simulink model "kopter_se_zavazim_state_feedback"  (R2024b)
settings: Solver=ode4  StartTime=0.0  StopTime=16  FixedStep=0.01  RelTol=1e-3
values from neighbouring files (symbols this model uses):
  b_moment = 3.6e-7    (= 3.6e-07)    [parametry_kopter_se_zavazim.m]
  d = 1    [parametry_kopter_se_zavazim.m]
  g = 9.81    [parametry_kopter_se_zavazim.m]
  init_int_dref = -Ki\((Uinit-Us)+Kp*(Xinit_ss-Xs))    [odvozeni_stavova_regulace_a_LQR.m]
  init_int_ref = -Ki\(Kp*xss+uss)    [odvozeni_stavova_regulace_a_LQR.m]
  Ip = m*d^2    (= 1)    [parametry_kopter_se_zavazim.m]
  Ixx = 0.0222    [parametry_kopter_se_zavazim.m]
  Iyy = 0.0222    [parametry_kopter_se_zavazim.m]
  Izz = 0.0429    [parametry_kopter_se_zavazim.m]
  k_thrust = 9.3e-6    (= 9.3e-06)    [parametry_kopter_se_zavazim.m]
  Ki = K_ex_other_angles(:, 17:20)    [odvozeni_stavova_regulace_a_LQR.m]
  Kp = K_ex_other_angles(:, 1:16)    [odvozeni_stavova_regulace_a_LQR.m]
  l = 0.2051    [parametry_kopter_se_zavazim.m]
  L_obs = place(Ac', Cc', poles_obs)'    [odvozeni_stavova_regulace_a_LQR.m]
  M = 2    [parametry_kopter_se_zavazim.m]
  m = 1    [parametry_kopter_se_zavazim.m]
  Us = [(M+m)*g; 0; 0; 0]    [parametry_kopter_se_zavazim.m]
  Xinit_ss = [Xinit_matrix; [0 0 0 0 0 0 0 0]']    [parametry_kopter_se_zavazim.m]
  Xs = [0;0;0; 0;0;0; 0;0; 0;0;0; 0;0;0; 0;0]    [parametry_kopter_se_zavazim.m]
undefined symbols (not defined in the file or in its folder): L
libraries: simulink_extras x16
(part 1 of 4)
settings Model: Creator=Admin  LastModifiedBy=Admin

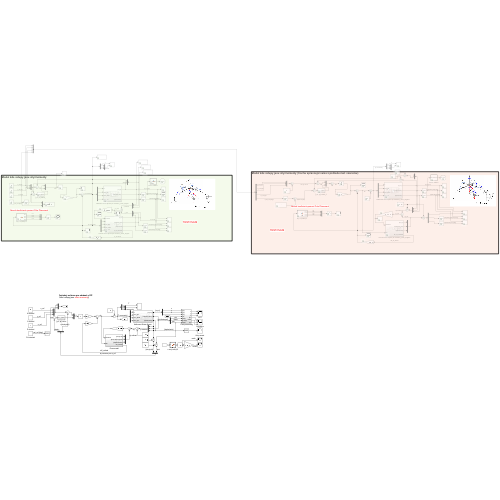
[thumbnail: Simulink's stored preview of the top-level diagram]
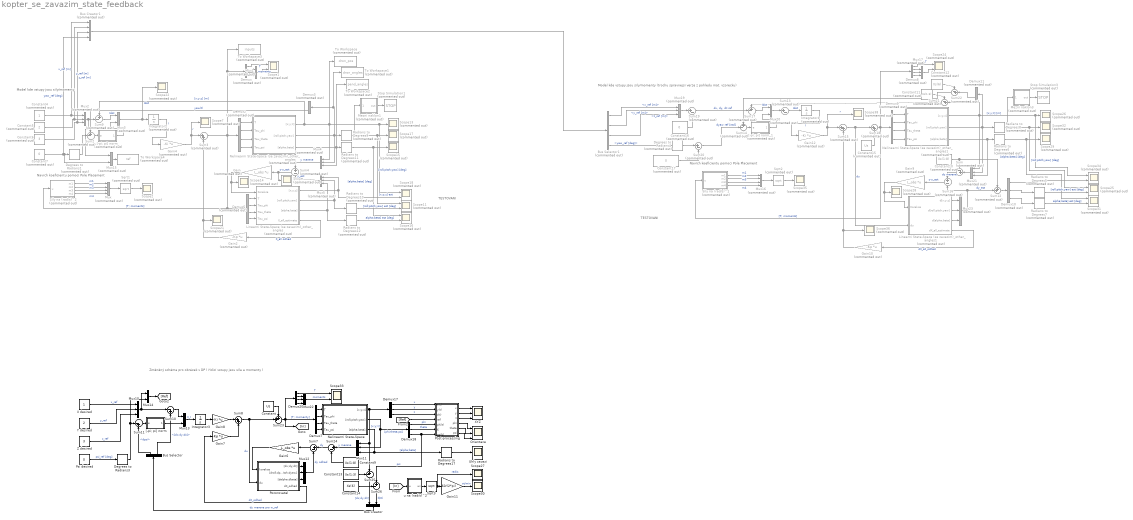
== system kopter_se_zavazim_state_feedback ==
  note: TESTOVANI
  note: Model kde vstupy jsou sily/momenty
  note: Navrch koeficientu pomoci Pole Placement
  note: Změněný schéma pro obrázek v DP
      | ( řídicí vstupy jsou síla a momenty )
  note: Model kde vstupy jsou sily/momenty (trochu spravnejsi verze z pohledu mat. vzorecku)
  note: Navrch koeficientu pomoci Pole Placement
  note: TESTOVANI
  Bus Creator : BusCreator  Inputs=2
  Bus Creator1 : BusCreator  Commented=on  Inputs=4
  Bus Selector : BusSelector  OutputSignals=dpsi,[dx;dy;dz]
  Bus Selector1 : BusSelector  Commented=on  OutputSignals=x_ref [m],y_ref [m],z_ref [m],yaw_ref [deg]
  Constant : Constant  Value=Us
  Constant10 : Constant  Commented=on  Value=Xs(1:8)
  Constant11 : Constant  Commented=on  Value=Xs(1:3)
  Constant12 : Constant  Commented=on  Value=Xs(6)
  Constant13 : Constant  Value=Xs(1:3)
  Constant14 : Constant  Value=Xs(6)
  Constant15 : Constant  Commented=on  Value=Us
  Constant16 : Constant  Commented=on  Value=0
  Constant17 : Constant  Commented=on  Value=0
  Constant4 : Constant  Commented=on
  Constant5 : Constant  Commented=on  Value=2
  Constant6 : Constant  Commented=on  Value=3
  Constant7 : Constant  Commented=on  Value=0
  Constant9 : Constant  Value=Xs(1:8)
  Degrees to Radians1 : simulink_extras/Transformations/Degrees to Radians  Commented=on
  Degrees to Radians3 : simulink_extras/Transformations/Degrees to Radians
  Degrees to Radians4 : simulink_extras/Transformations/Degrees to Radians  Commented=on
  Demux{,2,5,8..9} (5 alike) : Demux  Commented=on
  Demux10 : Demux  Commented=on  Outputs=3
  Demux11 : Demux  Commented=on  Outputs=3
  Demux17 : Demux  Outputs=3
  Demux18 : Demux  Outputs=3
  Demux20 : Demux
  Demux3 : Demux  Commented=on  Outputs=3
  Demux7 : Demux
  Gain : Gain  Commented=on  Gain=L_obs  Multiplication=Matrix(K*u)
  Gain10 : Gain  Commented=on  Gain=-Kp  Multiplication=Matrix(K*u)
  Gain11 : Gain  Gain=60/(2*pi)
  Gain12 : Gain  Commented=on  Gain=-Ki  Multiplication=Matrix(K*u)
  Gain2 : Gain  Commented=on  Gain=-Kp  Multiplication=Matrix(K*u)
  Gain4 : Gain  Commented=on  Gain=-Ki  Multiplication=Matrix(K*u)
  Gain6 : Gain  Gain=L_obs  Multiplication=Matrix(K*u)
  Gain7 : Gain  Gain=-Kp  Multiplication=Matrix(K*u)
  Gain8 : Gain  Gain=-Ki  Multiplication=Matrix(K*u)
  Gain9 : Gain  Commented=on  Gain=L_obs  Multiplication=Matrix(K*u)
  Integrator1 : Integrator  Commented=on  InitialCondition=init_int_ref
  Integrator3 : Integrator  InitialCondition=init_int_dref
  Integrator4 : Integrator  Commented=on  InitialCondition=init_int_dref
  Linearni State-Space (se zavazim)_other_angles : Subsystem  Commented=on
  Linearni State-Space (se zavazim)_other_angles1 : Subsystem  Commented=on
  Mezni naklon1 : MATLAB Function  Commented=on  TreatAsAtomicUnit=on
  Mezni naklon3 : MATLAB Function  Commented=on  TreatAsAtomicUnit=on
  Mux : Mux  Commented=on
  Mux{1..2,4..5,17,19,21,23} (8 alike) : Mux  Commented=on  Inputs=3
  Mux{10..12,22} (4 alike) : Mux  Inputs=3
  Mux13 : Mux  Inputs=2
  Mux14 : Mux  Inputs=2
  Mux15 : Mux  Commented=on  Inputs=2
  Mux16 : Mux  Commented=on
  Mux20 : Mux  Commented=on  Inputs=2
  Mux3 : Mux  Commented=on  Inputs=2
  Nelinearni State-Space : Subsystem
  Nelinearni State-Space (se zavazim)_other_angles : Subsystem  Commented=on
  Nelinearni State-Space (se zavazim)_other_angles1 : Subsystem  Commented=on
  Orientace : Scope  NumInputPorts=3
  Post-processing : Subsystem
  Pozorovatel : Subsystem
  Psi desired : Constant  Value=0
  Radians to Degrees{5..12} (8 alike) : simulink_extras/Transformations/Radians to Degrees  Commented=on
  Radians to Degrees17 : simulink_extras/Transformations/Radians to Degrees
  Scope{,2,7,13..15,17,21..22,26,28..29,32,35..36,38} (16 alike) : Scope  Commented=on
  Scope{1,11,16,18,24..25,31,34} (8 alike) : Scope  Commented=on  NumInputPorts=2
  Scope27 : Scope
  Scope30 : Scope
  Scope33 : Scope  NumInputPorts=2
  Sily na (rad/s)^1 : MATLAB Function  Commented=on  TreatAsAtomicUnit=on
  Sily na (rad/s)^2 : MATLAB Function  Commented=on  TreatAsAtomicUnit=on
  Sqrt1 : Sqrt  Commented=on
  Sqrt2 : Sqrt  Commented=on
  Sqrt3 : Sqrt
  Stop Simulation1 : Stop  Commented=on
  Stop Simulation3 : Stop  Commented=on
  Sum : Sum  Commented=on  Inputs=-+|
  Sum10 : Sum  Inputs=|-+
  Sum11 : Sum  Inputs=|-+
  Sum12 : Sum  Commented=on  Inputs=++|
  Sum13 : Sum  Commented=on  Inputs=|+-
  Sum{2,9,14,17} (4 alike) : Sum  Commented=on  Inputs=+-|
  Sum15 : Sum  Commented=on  Inputs=|++
  Sum16 : Sum  Commented=on  Inputs=+|-
  Sum18 : Sum  Commented=on  Inputs=|++
  Sum19 : Sum  Commented=on  Inputs=|+-
  Sum20 : Sum  Commented=on  Inputs=|+-
  Sum21 : Sum  Commented=on  Inputs=-+|
  Sum22 : Sum  Commented=on  Inputs=-+|
  Sum23 : Sum  Inputs=++|
  Sum24 : Sum  Inputs=|+-
  Sum25 : Sum  Inputs=-+|
  Sum26 : Sum  Inputs=-+|
  Sum3 : Sum  Commented=on  Inputs=|++
  Sum4 : Sum  Commented=on  Inputs=+|-
  Sum7 : Sum  Inputs=|+-
  Sum8 : Sum  Inputs=|++
  To Workspace : ToWorkspace  Commented=on  VariableName=dron_pos  SaveFormat=Timeseries  SampleTime=-1
  To Workspace1 : ToWorkspace  Commented=on  VariableName=dron_angles  SaveFormat=Timeseries  SampleTime=-1
  To Workspace2 : ToWorkspace  Commented=on  VariableName=pend_angles  SaveFormat=Timeseries  SampleTime=-1
  To Workspace3 : ToWorkspace  Commented=on  VariableName=inputs  SaveFormat=Timeseries  SampleTime=-1
  To Workspace4 : ToWorkspace  Commented=on  VariableName=ref  SaveFormat=Timeseries  SampleTime=-1
  Uhly zavazi : Scope
  X desired : Constant
  XYZ : Scope  NumInputPorts=3
  Y desired : Constant  Value=2
  Z desired : Constant  Value=3
  "[-pi; pi] norm" : Subsystem
  "[-pi; pi] norm_" : Subsystem  Commented=on
  "[-pi; pi] norm_1" : Subsystem  Commented=on
  u na (rad/s)^2 : MATLAB Function  TreatAsAtomicUnit=on
  wires:
  Linearni State-Space (se zavazim)_other_angles/1("[x;y;z]") -> Mux5/1, Scope18/2  "[x;y;z] est"
  Demux5/3 -> Linearni State-Space (se zavazim)_other_angles/4(Tau_theta)
  Demux5/2 -> Linearni State-Space (se zavazim)_other_angles/3(Tau_phi)
  Nelinearni State-Space (se zavazim)_other_angles/3("[alpha;beta]") -> To Workspace2/1, Mux4/3, Radians to Degrees11/1
  Linearni State-Space (se zavazim)_other_angles/3("[alpha;beta]") -> Radians to Degrees12/1, Mux5/3
  Radians to Degrees10/1 -> Scope11/2  "[roll;pitch;yaw] est [deg]"
  Linearni State-Space (se zavazim)_other_angles/2("[roll;pitch;yaw]") -> Mux5/2, Radians to Degrees10/1
  Radians to Degrees12/1 -> Scope16/2  "alpha;beta] est [deg]"
  Demux5/1 -> Linearni State-Space (se zavazim)_other_angles/2(T)
  Demux5/4 -> Linearni State-Space (se zavazim)_other_angles/5(Tau_psi)
  Radians to Degrees9/1 -> Scope11/1, Scope17/1, Mezni naklon1/1(angles)  "[roll;pitch;yaw] [deg]"
  Radians to Degrees11/1 -> Scope16/1, Scope15/1  "[alpha;beta] [deg]"
  Demux2/3 -> Nelinearni State-Space (se zavazim)_other_angles/3(Tau_theta)
  Demux2/2 -> Nelinearni State-Space (se zavazim)_other_angles/2(Tau_phi)
  Constant5/1 -> Bus Creator1/2, Mux2/2  "y_ref [m]"
  Constant7/1 -> Bus Creator1/4, Mux15/2, Degrees to Radians1/1  "yaw_ref [deg]"
  Constant6/1 -> Bus Creator1/3, Mux2/3  "z_ref [m]"
  Gain2/1 -> Scope21/1, Sum3/2
  Degrees to Radians1/1 -> Sum2/2
  Sum3/1 -> Sily na (rad/s)^2/1(u), Demux5/1, To Workspace3/1, Demux/1, Demux2/1  "[T; moments]"
  Demux2/4 -> Nelinearni State-Space (se zavazim)_other_angles/4(Tau_psi)
  Gain4/1 -> Scope7/1, Sum3/1  "r"
  Demux2/1 -> Nelinearni State-Space (se zavazim)_other_angles/1(T)
  Integrator1/1 -> Gain4/1  "I"
  Constant4/1 -> Bus Creator1/1, Mux2/1  "x_ref [m]"
  Demux3/3 -> Sum2/1  "yaw(t)"
  Nelinearni State-Space (se zavazim)_other_angles/1("[x;y;z]") -> Sum9/1, To Workspace/1, Mux4/1, Scope18/1, Scope13/1  "[x;y;z] [m]"
  Nelinearni State-Space (se zavazim)_other_angles/2("[roll;pitch;yaw]") -> To Workspace1/1, Demux3/1, Radians to Degrees9/1, Mux4/2
  Mezni naklon1/1(out) -> Stop Simulation1/1
  Linearni State-Space (se zavazim)_other_angles/4(X_all_estimate) -> Gain2/1  "X_all odhad"
  Gain/1 -> Scope14/1, Linearni State-Space (se zavazim)_other_angles/1(Korekce)
  Sum4/1 -> Scope/1, Gain/1  "y-y_est"
  Mux5/1 -> Sum4/2  "y_est"
  Sily na (rad/s)^2/4(m4) -> Mux/4  "m4"
  Sily na (rad/s)^2/2(m2) -> Mux/2  "m2"
  Sily na (rad/s)^2/1(m1) -> Mux/1  "m1"
  Sily na (rad/s)^2/3(m3) -> Mux/3  "m3"
  Mux/1 -> Sqrt1/1
  Mux4/1 -> Sum4/1  "y merene"
  Demux/1 -> Scope1/1  "T"
  Demux/2 -> Mux1/1
  Demux/3 -> Mux1/2
  Demux/4 -> Mux1/3
  Mux1/1 -> Scope1/2  "moments"
  X desired/1 -> Mux10/1  "x_ref"
  Y desired/1 -> Mux10/2  "y_ref"
  Z desired/1 -> Mux10/3  "z_ref"
  Psi desired/1 -> Degrees to Radians3/1  "psi_ref [deg]"
  Degrees to Radians3/1 -> Mux14/2, Sum11/1
  Demux7/1 -> Nelinearni State-Space/1(T)
  Demux7/2 -> Nelinearni State-Space/2(Tau_phi)
  Demux7/3 -> Nelinearni State-Space/3(Tau_theta)
  Demux7/4 -> Nelinearni State-Space/4(Tau_psi)
  Nelinearni State-Space/2("[roll;pitch;yaw]") -> Demux18/1, Mux11/2  "[phi;theta;psi]"
  Demux17/2 -> Post-processing/2(y(t))  "y"
  Nelinearni State-Space/1("[x;y;z]") -> Demux17/1, Sum25/2, Mux11/1  "[x;y;z]"
  Demux17/3 -> Post-processing/3(z(t))  "z"
  Nelinearni State-Space/3("[alpha;beta]") -> Radians to Degrees17/1, Mux11/3  "[alpha;beta]"
  Post-processing/3(z) -> XYZ/3
  Post-processing/2(y) -> XYZ/2
  Post-processing/1(x) -> XYZ/1
  Demux18/2 -> Post-processing/6(theta(t))  "theta"
  Radians to Degrees17/1 -> Uhly zavazi/1
  [Ref] -> Post-processing/4(ref)
  Post-processing/6(psi) -> Orientace/3
  Demux18/1 -> Post-processing/5(phi(t))  "phi"
  Demux18/3 -> Post-processing/7(psi(t)), Sum26/2  "psi"
  Post-processing/4(phi) -> Orientace/1
  Post-processing/5(theta) -> Orientace/2
  Demux17/1 -> Post-processing/1(x(t))  "x"
  Mux11/1 -> Sum24/1  "y merene"
  Pozorovatel/1("[dx;dy;dz]") -> Mux12/1
  Pozorovatel/2("[droll;dpitch;dyaw]") -> Mux12/2
  Pozorovatel/3("[dalpha;dbeta]") -> Mux12/3
  Mux12/1 -> Sum7/2  "dy odhad"
  Sum7/1 -> Gain6/1
  Gain6/1 -> Pozorovatel/1(korekce)
  Sum23/1 -> [In], Demux7/1, Demux20/1  "[T; momenty]"
  Integrator3/1 -> Gain8/1
  Gain8/1 -> Sum8/1
  Pozorovatel/4(dX_odhad) -> Gain7/1  "dX_odhad"
  Gain7/1 -> Sum8/2
  Demux20/2 -> Mux22/1
  Demux20/3 -> Mux22/2
  Demux20/1 -> Scope33/1  "T"
  Mux22/1 -> Scope33/2  "moments"
  Demux20/4 -> Mux22/3
  Bus Creator/1 -> Bus Selector/1  "dy merene pro w_ref"
  Sqrt1/1 -> Scope2/1
  Bus Selector/2 -> Sum10/2  "<[dx;dy;dz]>"
  Bus Selector/1 -> Sum11/2  "<dpsi>"
  Sqrt3/1 -> Gain11/1, Scope27/1  "rad/s"
  Gain11/1 -> Scope30/1  "ot/min"
  u na (rad/s)^2/1(wi) -> Sqrt3/1
  [In] -> u na (rad/s)^2/1(u)
  Mux2/1 -> Mux15/1, Sum9/2
  Sum2/1 -> "[-pi; pi] norm_"/1(e)
  Sum9/1 -> Mux3/1  "Idot"
  "[-pi; pi] norm_"/1(e_norm) -> Mux3/2
  Mux10/1 -> Mux14/1, Sum10/1
  Sum11/1 -> "[-pi; pi] norm"/1(e)
  Sum10/1 -> Mux13/1
  "[-pi; pi] norm"/1(e_norm) -> Mux13/2
  Mux13/1 -> Integrator3/1  "X_I"
  Mux14/1 -> [Ref]
  Mux3/1 -> Scope22/1, Integrator1/1  "Idot"
  Mux15/1 -> To Workspace4/1
  Bus Selector1/2 -> Mux19/2  "<y_ref [m]>"
  Nelinearni State-Space (se zavazim)_other_angles1/2("[roll;pitch;yaw]") -> Demux11/1, Mux21/2, Radians to Degrees8/1
  Radians to Degrees8/1 -> Scope25/1, Scope32/1, Mezni naklon3/1(angles)  "[roll;pitch;yaw] [deg]"
  Mux23/1 -> Sum12/2, Sum16/2  "dy_est"
  Sqrt2/1 -> Scope35/1
  Bus Selector1/4 -> Degrees to Radians4/1  "<yaw_ref [deg]>"
  Sum16/1 -> Gain9/1  "y-y_est"
  Bus Selector1/1 -> Mux19/1  "<x_ref [m]>"
  Sum14/1 -> "[-pi; pi] norm_1"/1(e)
  Sily na (rad/s)^1/2(m2) -> Mux16/2  "m2"
  Radians to Degrees5/1 -> Scope25/2  "[roll;pitch;yaw] est [deg]"
  Mux19/1 -> Sum19/1
  Mux20/1 -> Sum13/1
  Degrees to Radians4/1 -> Sum20/1
  Nelinearni State-Space (se zavazim)_other_angles1/3("[alpha;beta]") -> Mux21/3, Radians to Degrees6/1
  Bus Selector1/3 -> Mux19/3  "<z_ref [m]>"
  Mux16/1 -> Sqrt2/1
  Sily na (rad/s)^1/1(m1) -> Mux16/1  "m1"
  Linearni State-Space (se zavazim)_other_angles1/1(d[x;y;z]) -> Mux23/1
  Linearni State-Space (se zavazim)_other_angles1/4(dX_all_estimate) -> Gain10/1  "dX_all_odhad"
  Radians to Degrees7/1 -> Scope31/2  "alpha;beta] est [deg]"
  Demux9/3 -> Nelinearni State-Space (se zavazim)_other_angles1/3(Tau_theta)
  Gain9/1 -> Scope28/1, Linearni State-Space (se zavazim)_other_angles1/1(Korekce)
  Radians to Degrees6/1 -> Scope31/1, Scope29/1  "[alpha;beta] [deg]"
  Integrator4/1 -> Gain12/1  "I"
  Demux9/2 -> Nelinearni State-Space (se zavazim)_other_angles1/2(Tau_phi)
  Mezni naklon3/1(out) -> Stop Simulation3/1
  "[-pi; pi] norm_1"/1(e_norm) -> Mux20/2
  Sily na (rad/s)^1/3(m3) -> Mux16/3  "m3"
  Gain12/1 -> Sum15/1, Scope38/1  "r"
  Sum/1 -> Sum16/1  "dy merene"
  Sum17/1 -> Mux20/1  "Idot"
  Linearni State-Space (se zavazim)_other_angles1/3(d[alpha;beta]) -> Mux23/3
  Sum13/1 -> Integrator4/1  "Idot"
  Demux9/1 -> Nelinearni State-Space (se zavazim)_other_angles1/1(T)
  Linearni State-Space (se zavazim)_other_angles1/2(d[roll;pitch;yaw]) -> Mux23/2
  Demux9/4 -> Nelinearni State-Space (se zavazim)_other_angles1/4(Tau_psi)
  Sily na (rad/s)^1/4(m4) -> Mux16/4  "m4"
  Constant15/1 -> Sum18/2
  Demux8/4 -> Mux17/3
  Mux17/1 -> Scope24/2
  Demux8/3 -> Mux17/2
  Demux8/1 -> Scope24/1  "T"
  Sum18/1 -> Demux8/1, Sily na (rad/s)^1/1(u), Demux9/1  "[T; moments]"
  Demux8/2 -> Mux17/1
  Gain10/1 -> Sum15/2, Scope36/1
  Sum15/1 -> Linearni State-Space (se zavazim)_other_angles1/2(du), Sum18/1  "du"
  Sum19/1 -> Sum17/2  "dx, dy, dz ref"
  Constant16/1 -> Sum19/2
  Constant17/1 -> Sum20/2
  Sum20/1 -> Sum14/2  "dyaw ref [rad]"
  Nelinearni State-Space (se zavazim)_other_angles1/1("[x;y;z]") -> Sum21/2, Mux21/1, Scope34/1, Scope26/1  "[x;y;z] [m]"
  Bus Creator1/1 -> Bus Selector1/1
  Mux21/1 -> Sum/2
  Constant10/1 -> Sum12/1, Sum/1
  Sum12/1 -> Demux10/1
  Demux10/1 -> Scope34/2
  Demux10/2 -> Radians to Degrees5/1
  Demux10/3 -> Radians to Degrees7/1
  Sum21/1 -> Sum17/1
  Constant11/1 -> Sum21/1
  Sum22/1 -> Sum14/1
  Constant12/1 -> Sum22/1
  Demux11/3 -> Sum22/2
  Sum8/1 -> Sum23/2, Pozorovatel/2(du)  "du"
  Constant/1 -> Sum23/1
  Sum24/1 -> Sum7/1  "dy"
  Constant9/1 -> Sum24/2
  Sum25/1 -> Bus Creator/1  "[dx;dy;dz]"
  Constant13/1 -> Sum25/1
  Sum26/1 -> Bus Creator/2  "dpsi"
  Constant14/1 -> Sum26/1

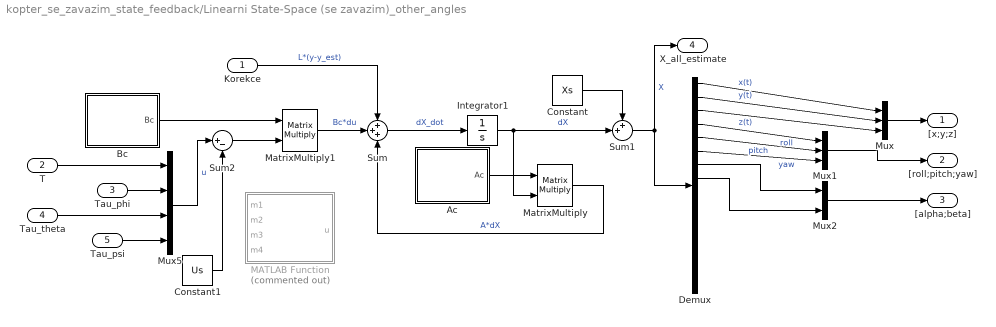
== system kopter_se_zavazim_state_feedback/Linearni State-Space (se zavazim)_other_angles ==
  Korekce : Inport
  T : Inport  Port=2
  Tau_phi : Inport  Port=3
  Tau_theta : Inport  Port=4
  Tau_psi : Inport  Port=5
  Ac : MATLAB Function  TreatAsAtomicUnit=on
  Bc : MATLAB Function  TreatAsAtomicUnit=on
  Constant : Constant  Value=Xs
  Constant1 : Constant  Value=Us
  Demux : Demux  Outputs=16
  Integrator1 : Integrator  InitialCondition=Xinit_ss - Xs
  MATLAB Function : MATLAB Function  Commented=on  TreatAsAtomicUnit=on
  MatrixMultiply : Product  Multiplication=Matrix(*)
  MatrixMultiply1 : Product  Multiplication=Matrix(*)
  Mux : Mux  Inputs=3
  Mux1 : Mux  Inputs=3
  Mux2 : Mux  Inputs=2
  Mux5 : Mux
  Sum : Sum  Inputs=+++
  Sum1 : Sum  Inputs=++|
  Sum2 : Sum  Inputs=|+-
  "[x;y;z]" : Outport
  "[roll;pitch;yaw]" : Outport  Port=2
  "[alpha;beta]" : Outport  Port=3
  X_all_estimate : Outport  Port=4
  wires:
  Mux5/1 -> Sum2/1  "u"
  Ac/1(Ac) -> MatrixMultiply/1
  Integrator1/1 -> Sum1/2, MatrixMultiply/2  "dX"
  Demux/1 -> Mux/1  "x(t)"
  Demux/2 -> Mux/2  "y(t)"
  Demux/3 -> Mux/3  "z(t)"
  Mux/1 -> "[x;y;z]"/1
  Demux/4 -> Mux1/1  "roll"
  Demux/5 -> Mux1/2  "pitch"
  Demux/6 -> Mux1/3  "yaw"
  Mux1/1 -> "[roll;pitch;yaw]"/1
  Sum/1 -> Integrator1/1  "dX_dot"
  MatrixMultiply1/1 -> Sum/2  "Bc*du"
  MatrixMultiply/1 -> Sum/3  "A*dX"
  Bc/1(Bc) -> MatrixMultiply1/1
  Sum1/1 -> Demux/1, X_all_estimate/1  "X"
  Constant/1 -> Sum1/1
  Constant1/1 -> Sum2/2
  Sum2/1 -> MatrixMultiply1/2
  Mux2/1 -> "[alpha;beta]"/1
  Demux/7 -> Mux2/1
  Demux/8 -> Mux2/2
  Tau_psi/1 -> Mux5/4
  T/1 -> Mux5/1
  Tau_theta/1 -> Mux5/3
  Tau_phi/1 -> Mux5/2
  Korekce/1 -> Sum/1  "L*(y-y_est)"

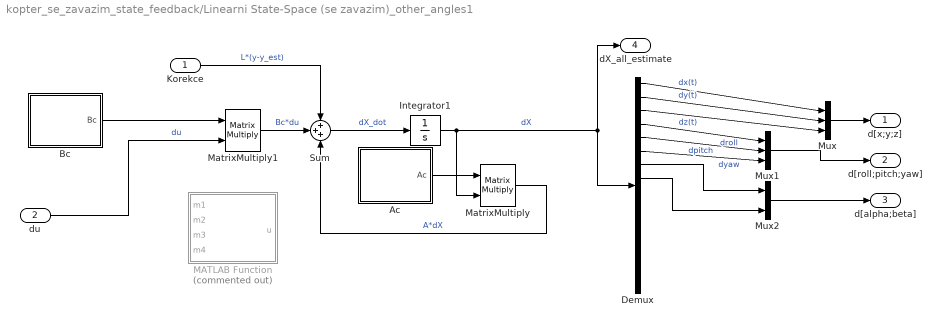
== system kopter_se_zavazim_state_feedback/Linearni State-Space (se zavazim)_other_angles1 ==
  Korekce : Inport
  du : Inport  Port=2
  Ac : MATLAB Function  TreatAsAtomicUnit=on
  Bc : MATLAB Function  TreatAsAtomicUnit=on
  Demux : Demux  Outputs=16
  Integrator1 : Integrator  InitialCondition=Xinit_ss - Xs
  MATLAB Function : MATLAB Function  Commented=on  TreatAsAtomicUnit=on
  MatrixMultiply : Product  Multiplication=Matrix(*)
  MatrixMultiply1 : Product  Multiplication=Matrix(*)
  Mux : Mux  Inputs=3
  Mux1 : Mux  Inputs=3
  Mux2 : Mux  Inputs=2
  Sum : Sum  Inputs=+++
  d[x;y;z] : Outport
  d[roll;pitch;yaw] : Outport  Port=2
  d[alpha;beta] : Outport  Port=3
  dX_all_estimate : Outport  Port=4
  wires:
  du/1 -> MatrixMultiply1/2  "du"
  Ac/1(Ac) -> MatrixMultiply/1
  Integrator1/1 -> Demux/1, dX_all_estimate/1, MatrixMultiply/2  "dX"
  Demux/1 -> Mux/1  "dx(t)"
  Demux/2 -> Mux/2  "dy(t)"
  Demux/3 -> Mux/3  "dz(t)"
  Mux/1 -> d[x;y;z]/1
  Demux/4 -> Mux1/1  "droll"
  Demux/5 -> Mux1/2  "dpitch"
  Demux/6 -> Mux1/3  "dyaw"
  Mux1/1 -> d[roll;pitch;yaw]/1
  Sum/1 -> Integrator1/1  "dX_dot"
  MatrixMultiply1/1 -> Sum/2  "Bc*du"
  MatrixMultiply/1 -> Sum/3  "A*dX"
  Bc/1(Bc) -> MatrixMultiply1/1
  Mux2/1 -> d[alpha;beta]/1
  Demux/7 -> Mux2/1
  Demux/8 -> Mux2/2
  Korekce/1 -> Sum/1  "L*(y-y_est)"

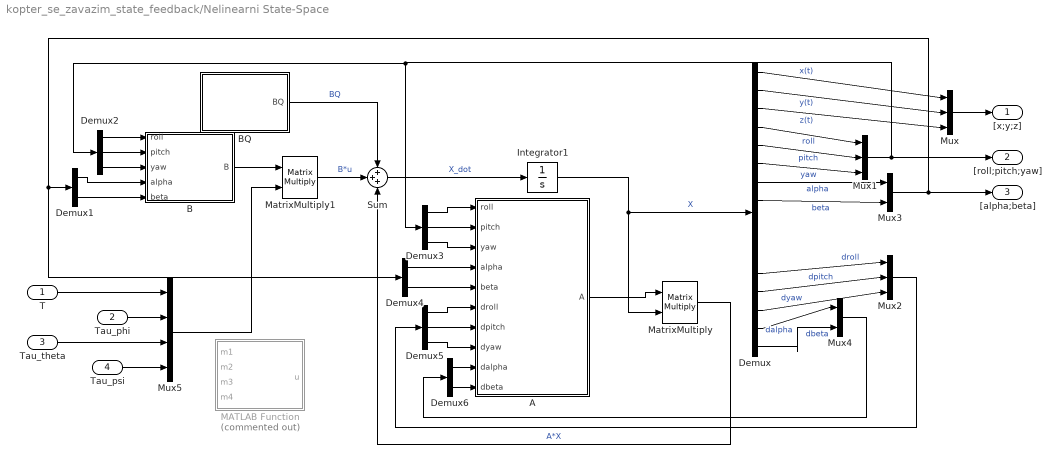
== system kopter_se_zavazim_state_feedback/Nelinearni State-Space ==
  T : Inport
  Tau_phi : Inport  Port=2
  Tau_theta : Inport  Port=3
  Tau_psi : Inport  Port=4
  A : MATLAB Function  TreatAsAtomicUnit=on
  B : MATLAB Function  TreatAsAtomicUnit=on
  BQ : MATLAB Function  TreatAsAtomicUnit=on
  Demux : Demux  Outputs=16
  Demux1 : Demux  Outputs=2
  Demux2 : Demux  Outputs=3
  Demux3 : Demux  Outputs=3
  Demux4 : Demux  Outputs=2
  Demux5 : Demux  Outputs=3
  Demux6 : Demux  Outputs=2
  Integrator1 : Integrator  InitialCondition=Xinit_ss
  MATLAB Function : MATLAB Function  Commented=on  TreatAsAtomicUnit=on
  MatrixMultiply : Product  Multiplication=Matrix(*)
  MatrixMultiply1 : Product  Multiplication=Matrix(*)
  Mux : Mux  Inputs=3
  Mux1 : Mux  Inputs=3
  Mux2 : Mux  Inputs=3
  Mux3 : Mux  Inputs=2
  Mux4 : Mux  Inputs=2
  Mux5 : Mux
  Sum : Sum  Inputs=+++
  "[x;y;z]" : Outport
  "[roll;pitch;yaw]" : Outport  Port=2
  "[alpha;beta]" : Outport  Port=3
  wires:
  A/1(A) -> MatrixMultiply/1
  Integrator1/1 -> MatrixMultiply/2, Demux/1  "X"
  Demux/1 -> Mux/1  "x(t)"
  Demux/2 -> Mux/2  "y(t)"
  Demux/3 -> Mux/3  "z(t)"
  Mux/1 -> "[x;y;z]"/1
  Demux/4 -> Mux1/1  "roll"
  Demux/5 -> Mux1/2  "pitch"
  Demux/6 -> Mux1/3  "yaw"
  Mux1/1 -> Demux2/1, Demux3/1, "[roll;pitch;yaw]"/1
  Demux/12 -> Mux2/1  "droll"
  Demux/13 -> Mux2/2  "dpitch"
  Demux/14 -> Mux2/3  "dyaw"
  Demux2/1 -> B/1(roll)
  Demux2/2 -> B/2(pitch)
  Demux2/3 -> B/3(yaw)
  Demux3/2 -> A/2(pitch)
  Demux3/1 -> A/1(roll)
  Demux3/3 -> A/3(yaw)
  Demux5/2 -> A/7(dpitch)
  Demux5/1 -> A/6(droll)
  Demux5/3 -> A/8(dyaw)
  Sum/1 -> Integrator1/1  "X_dot"
  BQ/1(BQ) -> Sum/1  "BQ"
  MatrixMultiply1/1 -> Sum/2  "B*u"
  B/1(B) -> MatrixMultiply1/1
  MatrixMultiply/1 -> Sum/3  "A*X"
  Mux2/1 -> Demux5/1
  Demux/7 -> Mux3/1  "alpha"
  Demux/8 -> Mux3/2  "beta"
  Mux3/1 -> Demux4/1, Demux1/1, "[alpha;beta]"/1
  Demux1/2 -> B/5(beta)
  Demux1/1 -> B/4(alpha)
  Demux4/2 -> A/5(beta)
  Demux4/1 -> A/4(alpha)
  Demux/15 -> Mux4/1  "dalpha"
  Demux/16 -> Mux4/2  "dbeta"
  Demux6/1 -> A/9(dalpha)
  Demux6/2 -> A/10(dbeta)
  Mux4/1 -> Demux6/1
  Tau_theta/1 -> Mux5/3
  Tau_psi/1 -> Mux5/4
  Tau_phi/1 -> Mux5/2
  Mux5/1 -> MatrixMultiply1/2
  T/1 -> Mux5/1

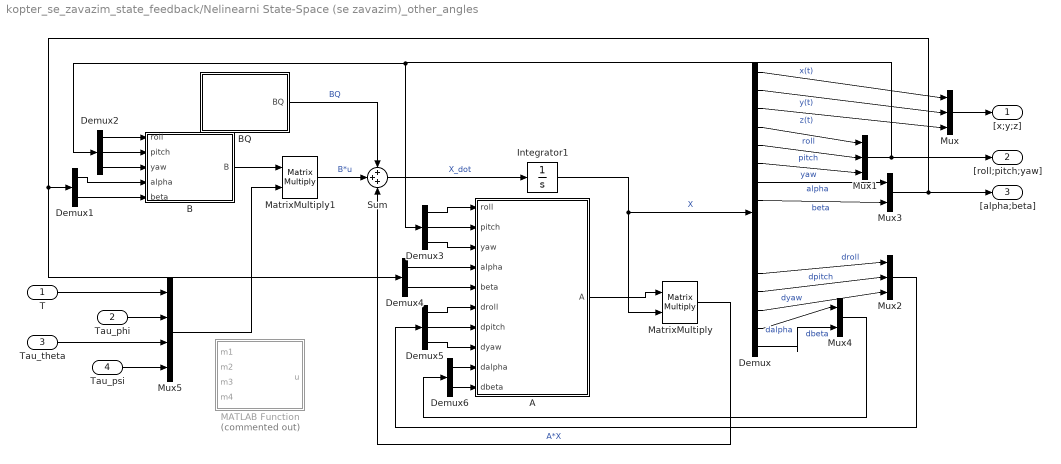
== system kopter_se_zavazim_state_feedback/Nelinearni State-Space (se zavazim)_other_angles ==
  T : Inport
  Tau_phi : Inport  Port=2
  Tau_theta : Inport  Port=3
  Tau_psi : Inport  Port=4
  A : MATLAB Function  TreatAsAtomicUnit=on
  B : MATLAB Function  TreatAsAtomicUnit=on
  BQ : MATLAB Function  TreatAsAtomicUnit=on
  Demux : Demux  Outputs=16
  Demux1 : Demux  Outputs=2
  Demux2 : Demux  Outputs=3
  Demux3 : Demux  Outputs=3
  Demux4 : Demux  Outputs=2
  Demux5 : Demux  Outputs=3
  Demux6 : Demux  Outputs=2
  Integrator1 : Integrator  InitialCondition=Xinit_ss
  MATLAB Function : MATLAB Function  Commented=on  TreatAsAtomicUnit=on
  MatrixMultiply : Product  Multiplication=Matrix(*)
  MatrixMultiply1 : Product  Multiplication=Matrix(*)
  Mux : Mux  Inputs=3
  Mux1 : Mux  Inputs=3
  Mux2 : Mux  Inputs=3
  Mux3 : Mux  Inputs=2
  Mux4 : Mux  Inputs=2
  Mux5 : Mux
  Sum : Sum  Inputs=+++
  "[x;y;z]" : Outport
  "[roll;pitch;yaw]" : Outport  Port=2
  "[alpha;beta]" : Outport  Port=3
  wires:
  A/1(A) -> MatrixMultiply/1
  Integrator1/1 -> MatrixMultiply/2, Demux/1  "X"
  Demux/1 -> Mux/1  "x(t)"
  Demux/2 -> Mux/2  "y(t)"
  Demux/3 -> Mux/3  "z(t)"
  Mux/1 -> "[x;y;z]"/1
  Demux/4 -> Mux1/1  "roll"
  Demux/5 -> Mux1/2  "pitch"
  Demux/6 -> Mux1/3  "yaw"
  Mux1/1 -> Demux2/1, Demux3/1, "[roll;pitch;yaw]"/1
  Demux/12 -> Mux2/1  "droll"
  Demux/13 -> Mux2/2  "dpitch"
  Demux/14 -> Mux2/3  "dyaw"
  Demux2/1 -> B/1(roll)
  Demux2/2 -> B/2(pitch)
  Demux2/3 -> B/3(yaw)
  Demux3/2 -> A/2(pitch)
  Demux3/1 -> A/1(roll)
  Demux3/3 -> A/3(yaw)
  Demux5/2 -> A/7(dpitch)
  Demux5/1 -> A/6(droll)
  Demux5/3 -> A/8(dyaw)
  Sum/1 -> Integrator1/1  "X_dot"
  BQ/1(BQ) -> Sum/1  "BQ"
  MatrixMultiply1/1 -> Sum/2  "B*u"
  B/1(B) -> MatrixMultiply1/1
  MatrixMultiply/1 -> Sum/3  "A*X"
  Mux2/1 -> Demux5/1
  Demux/7 -> Mux3/1  "alpha"
  Demux/8 -> Mux3/2  "beta"
  Mux3/1 -> Demux4/1, Demux1/1, "[alpha;beta]"/1
  Demux1/2 -> B/5(beta)
  Demux1/1 -> B/4(alpha)
  Demux4/2 -> A/5(beta)
  Demux4/1 -> A/4(alpha)
  Demux/15 -> Mux4/1  "dalpha"
  Demux/16 -> Mux4/2  "dbeta"
  Demux6/1 -> A/9(dalpha)
  Demux6/2 -> A/10(dbeta)
  Mux4/1 -> Demux6/1
  Tau_theta/1 -> Mux5/3
  Tau_psi/1 -> Mux5/4
  Tau_phi/1 -> Mux5/2
  Mux5/1 -> MatrixMultiply1/2
  T/1 -> Mux5/1

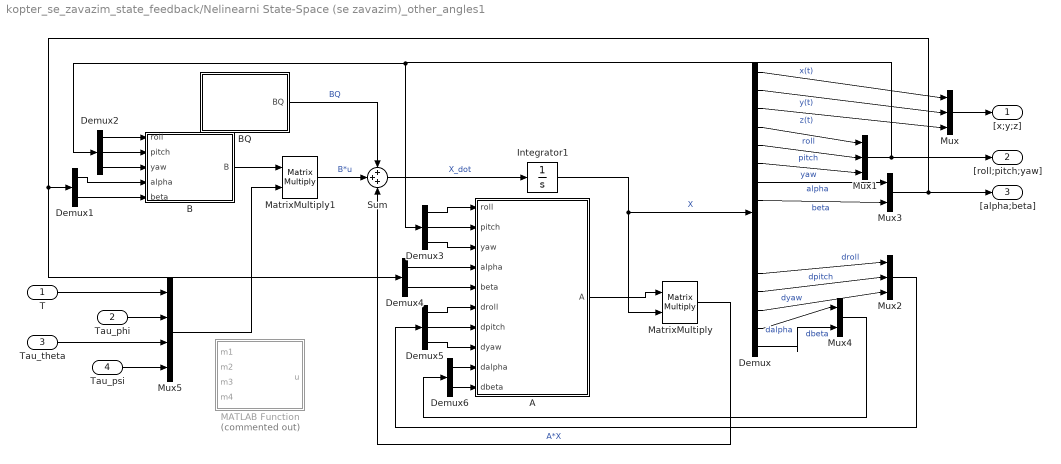
== system kopter_se_zavazim_state_feedback/Nelinearni State-Space (se zavazim)_other_angles1 ==
  T : Inport
  Tau_phi : Inport  Port=2
  Tau_theta : Inport  Port=3
  Tau_psi : Inport  Port=4
  A : MATLAB Function  TreatAsAtomicUnit=on
  B : MATLAB Function  TreatAsAtomicUnit=on
  BQ : MATLAB Function  TreatAsAtomicUnit=on
  Demux : Demux  Outputs=16
  Demux1 : Demux  Outputs=2
  Demux2 : Demux  Outputs=3
  Demux3 : Demux  Outputs=3
  Demux4 : Demux  Outputs=2
  Demux5 : Demux  Outputs=3
  Demux6 : Demux  Outputs=2
  Integrator1 : Integrator  InitialCondition=Xinit_ss
  MATLAB Function : MATLAB Function  Commented=on  TreatAsAtomicUnit=on
  MatrixMultiply : Product  Multiplication=Matrix(*)
  MatrixMultiply1 : Product  Multiplication=Matrix(*)
  Mux : Mux  Inputs=3
  Mux1 : Mux  Inputs=3
  Mux2 : Mux  Inputs=3
  Mux3 : Mux  Inputs=2
  Mux4 : Mux  Inputs=2
  Mux5 : Mux
  Sum : Sum  Inputs=+++
  "[x;y;z]" : Outport
  "[roll;pitch;yaw]" : Outport  Port=2
  "[alpha;beta]" : Outport  Port=3
  wires:
  A/1(A) -> MatrixMultiply/1
  Integrator1/1 -> MatrixMultiply/2, Demux/1  "X"
  Demux/1 -> Mux/1  "x(t)"
  Demux/2 -> Mux/2  "y(t)"
  Demux/3 -> Mux/3  "z(t)"
  Mux/1 -> "[x;y;z]"/1
  Demux/4 -> Mux1/1  "roll"
  Demux/5 -> Mux1/2  "pitch"
  Demux/6 -> Mux1/3  "yaw"
  Mux1/1 -> Demux2/1, Demux3/1, "[roll;pitch;yaw]"/1
  Demux/12 -> Mux2/1  "droll"
  Demux/13 -> Mux2/2  "dpitch"
  Demux/14 -> Mux2/3  "dyaw"
  Demux2/1 -> B/1(roll)
  Demux2/2 -> B/2(pitch)
  Demux2/3 -> B/3(yaw)
  Demux3/2 -> A/2(pitch)
  Demux3/1 -> A/1(roll)
  Demux3/3 -> A/3(yaw)
  Demux5/2 -> A/7(dpitch)
  Demux5/1 -> A/6(droll)
  Demux5/3 -> A/8(dyaw)
  Sum/1 -> Integrator1/1  "X_dot"
  BQ/1(BQ) -> Sum/1  "BQ"
  MatrixMultiply1/1 -> Sum/2  "B*u"
  B/1(B) -> MatrixMultiply1/1
  MatrixMultiply/1 -> Sum/3  "A*X"
  Mux2/1 -> Demux5/1
  Demux/7 -> Mux3/1  "alpha"
  Demux/8 -> Mux3/2  "beta"
  Mux3/1 -> Demux4/1, Demux1/1, "[alpha;beta]"/1
  Demux1/2 -> B/5(beta)
  Demux1/1 -> B/4(alpha)
  Demux4/2 -> A/5(beta)
  Demux4/1 -> A/4(alpha)
  Demux/15 -> Mux4/1  "dalpha"
  Demux/16 -> Mux4/2  "dbeta"
  Demux6/1 -> A/9(dalpha)
  Demux6/2 -> A/10(dbeta)
  Mux4/1 -> Demux6/1
  Tau_theta/1 -> Mux5/3
  Tau_psi/1 -> Mux5/4
  Tau_phi/1 -> Mux5/2
  Mux5/1 -> MatrixMultiply1/2
  T/1 -> Mux5/1

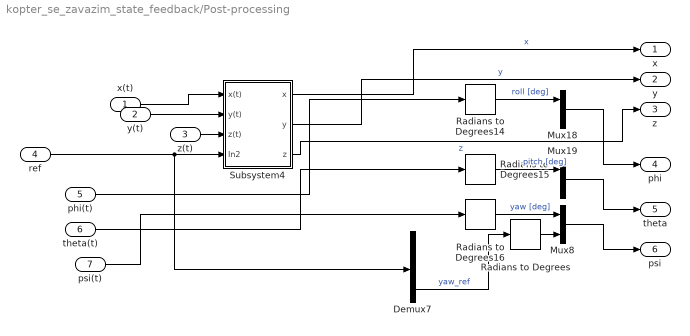
== system kopter_se_zavazim_state_feedback/Post-processing ==
  x(t) : Inport
  y(t) : Inport  Port=2
  z(t) : Inport  Port=3
  ref : Inport  Port=4
  phi(t) : Inport  Port=5
  theta(t) : Inport  Port=6
  psi(t) : Inport  Port=7
  Demux7 : Demux
  Mux18 : Mux  Inputs=2
  Mux19 : Mux  Inputs=2
  Mux8 : Mux  Inputs=2
  Radians to Degrees{,14..16} (4 alike) : simulink_extras/Transformations/Radians to Degrees
  Subsystem4 : Subsystem
  x : Outport
  y : Outport  Port=2
  z : Outport  Port=3
  phi : Outport  Port=4
  theta : Outport  Port=5
  psi : Outport  Port=6
  wires:
  Radians to Degrees16/1 -> Mux8/1  "yaw [deg]"
  ref/1 -> Subsystem4/4(In2), Demux7/1
  Demux7/4 -> Radians to Degrees/1  "yaw_ref"
  theta(t)/1 -> Radians to Degrees15/1
  Mux18/1 -> phi/1
  Subsystem4/3(z) -> z/1  "z"
  Radians to Degrees14/1 -> Mux18/1  "roll [deg]"
  Radians to Degrees15/1 -> Mux19/1  "pitch [deg]"
  Subsystem4/2(y) -> y/1  "y"
  x(t)/1 -> Subsystem4/1(x(t))
  y(t)/1 -> Subsystem4/2(y(t))
  psi(t)/1 -> Radians to Degrees16/1
  phi(t)/1 -> Radians to Degrees14/1
  Subsystem4/1(x) -> x/1  "x"
  Mux8/1 -> psi/1
  z(t)/1 -> Subsystem4/3(z(t))
  Mux19/1 -> theta/1
  Radians to Degrees/1 -> Mux8/2

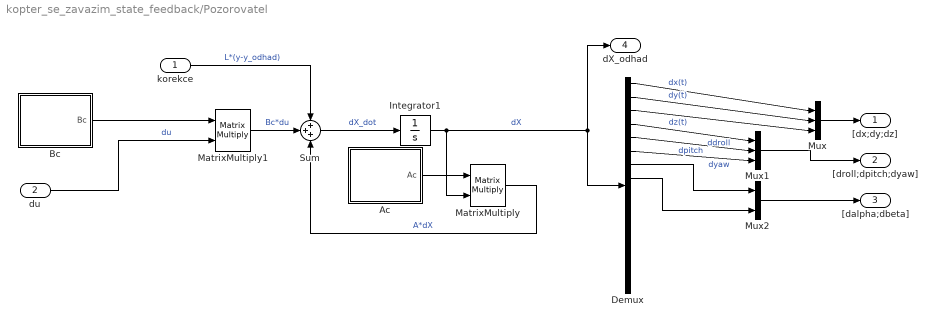
== system kopter_se_zavazim_state_feedback/Pozorovatel ==
  korekce : Inport
  du : Inport  Port=2
  Ac : MATLAB Function  TreatAsAtomicUnit=on
  Bc : MATLAB Function  TreatAsAtomicUnit=on
  Demux : Demux  Outputs=16
  Integrator1 : Integrator  InitialCondition=Xinit_ss - Xs
  MatrixMultiply : Product  Multiplication=Matrix(*)
  MatrixMultiply1 : Product  Multiplication=Matrix(*)
  Mux : Mux  Inputs=3
  Mux1 : Mux  Inputs=3
  Mux2 : Mux  Inputs=2
  Sum : Sum  Inputs=+++
  "[dx;dy;dz]" : Outport
  "[droll;dpitch;dyaw]" : Outport  Port=2
  "[dalpha;dbeta]" : Outport  Port=3
  dX_odhad : Outport  Port=4
  wires:
  du/1 -> MatrixMultiply1/2  "du"
  Ac/1(Ac) -> MatrixMultiply/1
  Integrator1/1 -> Demux/1, dX_odhad/1, MatrixMultiply/2  "dX"
  Demux/1 -> Mux/1  "dx(t)"
  Demux/2 -> Mux/2  "dy(t)"
  Demux/3 -> Mux/3  "dz(t)"
  Mux/1 -> "[dx;dy;dz]"/1
  Demux/4 -> Mux1/1  "ddroll"
  Demux/5 -> Mux1/2  "dpitch"
  Demux/6 -> Mux1/3  "dyaw"
  Mux1/1 -> "[droll;dpitch;dyaw]"/1
  Sum/1 -> Integrator1/1  "dX_dot"
  MatrixMultiply1/1 -> Sum/2  "Bc*du"
  MatrixMultiply/1 -> Sum/3  "A*dX"
  Bc/1(Bc) -> MatrixMultiply1/1
  Mux2/1 -> "[dalpha;dbeta]"/1
  Demux/7 -> Mux2/1
  Demux/8 -> Mux2/2
  korekce/1 -> Sum/1  "L*(y-y_odhad)"

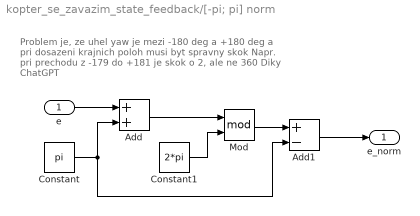
== system kopter_se_zavazim_state_feedback/[-pi; pi] norm ==
  note: Problem je, ze uhel yaw je mezi -180 deg a +180 deg
      | a pri dosazeni krajnich poloh musi byt spravny skok
      | Napr. pri prechodu z -179 do +181 je skok o 2, ale ne 360
      | Diky ChatGPT
  e : Inport
  Add : Sum
  Add1 : Sum  Inputs=+-
  Constant : Constant  Value=pi
  Constant1 : Constant  Value=2*pi
  Mod : Math  Operator=mod
  e_norm : Outport
  wires:
  e/1 -> Add/1
  Add/1 -> Mod/1
  Constant/1 -> Add1/2, Add/2
  Constant1/1 -> Mod/2
  Mod/1 -> Add1/1
  Add1/1 -> e_norm/1

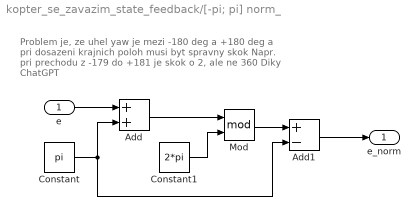
== system kopter_se_zavazim_state_feedback/[-pi; pi] norm_ ==
  note: Problem je, ze uhel yaw je mezi -180 deg a +180 deg
      | a pri dosazeni krajnich poloh musi byt spravny skok
      | Napr. pri prechodu z -179 do +181 je skok o 2, ale ne 360
      | Diky ChatGPT
  e : Inport
  Add : Sum
  Add1 : Sum  Inputs=+-
  Constant : Constant  Value=pi
  Constant1 : Constant  Value=2*pi
  Mod : Math  Operator=mod
  e_norm : Outport
  wires:
  e/1 -> Add/1
  Add/1 -> Mod/1
  Constant/1 -> Add1/2, Add/2
  Constant1/1 -> Mod/2
  Mod/1 -> Add1/1
  Add1/1 -> e_norm/1

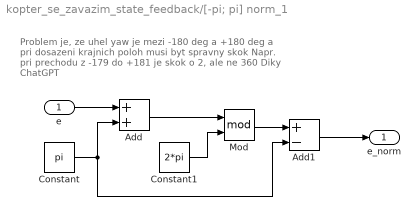
== system kopter_se_zavazim_state_feedback/[-pi; pi] norm_1 ==
  note: Problem je, ze uhel yaw je mezi -180 deg a +180 deg
      | a pri dosazeni krajnich poloh musi byt spravny skok
      | Napr. pri prechodu z -179 do +181 je skok o 2, ale ne 360
      | Diky ChatGPT
  e : Inport
  Add : Sum
  Add1 : Sum  Inputs=+-
  Constant : Constant  Value=pi
  Constant1 : Constant  Value=2*pi
  Mod : Math  Operator=mod
  e_norm : Outport
  wires:
  e/1 -> Add/1
  Add/1 -> Mod/1
  Constant/1 -> Add1/2, Add/2
  Constant1/1 -> Mod/2
  Mod/1 -> Add1/1
  Add1/1 -> e_norm/1

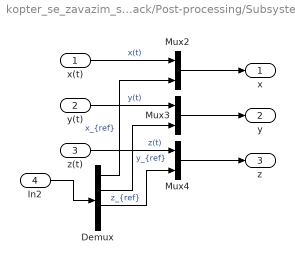
== system kopter_se_zavazim_state_feedback/Post-processing/Subsystem4 ==
  x(t) : Inport
  y(t) : Inport  Port=2
  z(t) : Inport  Port=3
  In2 : Inport  Port=4
  Demux : Demux
  Mux2 : Mux  Inputs=2
  Mux3 : Mux  Inputs=2
  Mux4 : Mux  Inputs=2
  x : Outport
  y : Outport  Port=2
  z : Outport  Port=3
  wires:
  Demux/2 -> Mux3/2  "y_{ref}"
  Mux4/1 -> z/1
  y(t)/1 -> Mux3/1  "y(t)"
  Mux3/1 -> y/1
  Demux/1 -> Mux2/2  "x_{ref}"
  Demux/3 -> Mux4/2  "z_{ref}"
  Mux2/1 -> x/1
  In2/1 -> Demux/1
  x(t)/1 -> Mux2/1  "x(t)"
  z(t)/1 -> Mux4/1  "z(t)"

== matlab function kopter_se_zavazim_state_feedback/Nelinearni State-Space/B ==
  data: roll input; B output; pitch input; yaw input; alpha input; beta input; M parameter; Ixx parameter; Iyy parameter; Izz parameter; Ip parameter; d parameter; m parameter
function B = fcn(roll, pitch, yaw, alpha, beta, M, Ixx, Iyy, Izz, Ip, d, m)
% Matice vstupu do soustavy kvadrokoptery se zavazim

phi_t = roll;
theta_t = pitch;
psi_t = yaw;

alpha_t = alpha;
beta_t = beta;

B = [ 
                                                                                                                                                                                                                                                                                                                                                                                                                                                                                                                                                                                   0,                                                                                                                                                                           0,                                                                        0,                                                                                          0;
                                                                                                                                                                                                                                                                                                                                                                                                                                                                                                                                                                                   0,                                                                                                                                                                           0,                                                                        0,                                                                                          0;
                                                                                                                                                                                                                                                                                                                                                                                                                                                                                                                                                                                   0,                                                                                                                                                                           0,                                                                        0,                                                                                          0;
                                                                                                                                                                                                                                                                                                                                                                                                                                                                                                                                                                                   0,                                                                                                                                                                           0,                                                                        0,                                                                                          0;
                                                                                                                                                                                                                                                                                                                                                                                                                                                                                                                                                                                   0,                                                                                                                                                                           0,                                                                        0,                                                                                          0;
                                                                                                                                                                                                                                                                                                                                                                                                                                                                                                                                                                                   0,                                                                                                                                                                           0,                                                                        0,                                                                                          0;
                                                                                                                                                                                                                                                                                                                                                                                                                                                                                                                                                                                   0,                                                                                                                                                                           0,                                                                        0,                                                                                          0;
                                                                                                                                                                                                                                                                                                                                                                                                                                                                                                                                                                                   0,                                                                                                                                                                           0,                                                                        0,                                                                                          0;
(M*sin(phi_t)*sin(psi_t) + m*sin(phi_t)*sin(psi_t) + M*cos(phi_t)*cos(psi_t)*sin(theta_t) + m*cos(phi_t)*cos(psi_t)*sin(theta_t) - m*cos(beta_t)^2*sin(phi_t)*sin(psi_t) - m*cos(beta_t)^2*cos(phi_t)*cos(psi_t)*sin(theta_t) + m*cos(alpha_t)^2*cos(beta_t)^2*sin(phi_t)*sin(psi_t) + m*cos(alpha_t)*cos(beta_t)^2*cos(phi_t)*sin(alpha_t)*cos(theta_t) + m*cos(alpha_t)^2*cos(beta_t)^2*cos(phi_t)*cos(psi_t)*sin(theta_t) + m*cos(beta_t)*cos(psi_t)*sin(alpha_t)*sin(beta_t)*sin(phi_t) - m*cos(beta_t)*cos(phi_t)*sin(alpha_t)*sin(beta_t)*sin(psi_t)*sin(theta_t))/(M*(M + m)),                                                                                                                                                                           0,                                                                        0,                                                                                          0;
                                                                                                                                                                                              -(M*cos(psi_t)*sin(phi_t) - M*cos(phi_t)*sin(psi_t)*sin(theta_t) + m*cos(beta_t)^2*cos(psi_t)*sin(phi_t) - m*cos(beta_t)^2*cos(phi_t)*sin(psi_t)*sin(theta_t) + m*cos(beta_t)*sin(alpha_t)*sin(beta_t)*sin(phi_t)*sin(psi_t) - m*cos(alpha_t)*cos(beta_t)*cos(phi_t)*sin(beta_t)*cos(theta_t) + m*cos(beta_t)*cos(phi_t)*cos(psi_t)*sin(alpha_t)*sin(beta_t)*sin(theta_t))/(M*(M + m)),                                                                                                                                                                           0,                                                                        0,                                                                                          0;
                                                                                                                                                            (M*cos(phi_t)*cos(theta_t) + m*cos(phi_t)*cos(theta_t) - m*cos(alpha_t)^2*cos(beta_t)^2*cos(phi_t)*cos(theta_t) + m*cos(alpha_t)*cos(beta_t)^2*sin(alpha_t)*sin(phi_t)*sin(psi_t) - m*cos(alpha_t)*cos(beta_t)*cos(psi_t)*sin(beta_t)*sin(phi_t) + m*cos(alpha_t)*cos(beta_t)^2*cos(phi_t)*cos(psi_t)*sin(alpha_t)*sin(theta_t) + m*cos(alpha_t)*cos(beta_t)*cos(phi_t)*sin(beta_t)*sin(psi_t)*sin(theta_t))/(M*(M + m)),                                                                                                                                                                           0,                                                                        0,                                                                                          0;
                                                                                                                                                                                                                                                                                                                                                                                                                                                                                                                                                                                   0, -(Iyy*Izz + Ixx*Iyy*sin(theta_t)^2 - Iyy*Izz*sin(theta_t)^2 - Ixx*Iyy*sin(phi_t)^2*sin(theta_t)^2 + Ixx*Izz*sin(phi_t)^2*sin(theta_t)^2)/(Ixx*Iyy*Izz*(sin(theta_t)^2 - 1)), -(cos(phi_t)*sin(phi_t)*sin(theta_t)*(Iyy - Izz))/(Iyy*Izz*cos(theta_t)), -(sin(theta_t)*(Iyy - Iyy*sin(phi_t)^2 + Izz*sin(phi_t)^2))/(Iyy*Izz*(sin(theta_t)^2 - 1));
                                                                                                                                                                                                                                                                                                                                                                                                                                                                                                                                                                                   0,                                                                                                    -(cos(phi_t)*sin(phi_t)*sin(theta_t)*(Iyy - Izz))/(Iyy*Izz*cos(theta_t)),                    (Izz + Iyy*sin(phi_t)^2 - Izz*sin(phi_t)^2)/(Iyy*Izz),                                       -(sin(2*phi_t)*(Iyy - Izz))/(2*Iyy*Izz*cos(theta_t));
                                                                                                                                                                                                                                                                                                                                                                                                                                                                                                                                                                                   0,                                                                                  -(sin(theta_t)*(Iyy - Iyy*sin(phi_t)^2 + Izz*sin(phi_t)^2))/(Iyy*Izz*(sin(theta_t)^2 - 1)),                     -(sin(2*phi_t)*(Iyy - Izz))/(2*Iyy*Izz*cos(theta_t)),                -(Iyy - Iyy*sin(phi_t)^2 + Izz*sin(phi_t)^2)/(Iyy*Izz*(sin(theta_t)^2 - 1));
                                                                                                                                                                                                                                                                                                                                                                                                                                    -(cos(phi_t)*sin(alpha_t)*cos(theta_t) + cos(alpha_t)*sin(phi_t)*sin(psi_t) + cos(alpha_t)*cos(phi_t)*cos(psi_t)*sin(theta_t))/(M*d*cos(beta_t)),                                                                                                                                                                           0,                                                                        0,                                                                                          0;
                                                                                                                                                                                                                                                                                                                        (cos(beta_t)*cos(psi_t)*sin(phi_t) - cos(alpha_t)*cos(phi_t)*sin(beta_t)*cos(theta_t) - cos(beta_t)*cos(phi_t)*sin(psi_t)*sin(theta_t) + sin(alpha_t)*sin(beta_t)*sin(phi_t)*sin(psi_t) + cos(phi_t)*cos(psi_t)*sin(alpha_t)*sin(beta_t)*sin(theta_t))/(M*d),                                                                                                                                                                           0,                                                                        0,                                                                                          0];

== matlab function kopter_se_zavazim_state_feedback/Nelinearni State-Space/BQ ==
  data: BQ output; g parameter
function BQ = fcn(g)
% Matice vstupu tihy
BQ = [0 0 0 0 0 0 0 0 0 0 -g 0 0 0 0 0]';

== matlab function kopter_se_zavazim_state_feedback/Nelinearni State-Space/MATLAB Function ==
  data: u output; m1 input; m2 input; m3 input; m4 input; k_thrust parameter; b_moment parameter; L parameter
function u = fcn(m1, m2, m3, m4, k_thrust, b_moment, L)

Thrust = k_thrust*(m1^2 + m2^2 + m3^2 + m4^2);
Tau_roll = L*k_thrust*(m1^2 + m4^2 - m2^2 - m3^2);
Tau_pitch = L*k_thrust*(m4^2 + m3^2 - m1^2 - m2^2);
Tau_yaw = b_moment*(m1^2 + m3^2 - m2^2 - m4^2);

u = [Thrust; Tau_roll; Tau_pitch; Tau_yaw];

== matlab function kopter_se_zavazim_state_feedback/Pozorovatel/Ac ==
  data: g parameter; M parameter; Ac output; m parameter; Ip parameter; d parameter
function Ac = fcn(g, M, m, Ip, d)
% Matice Ac linearizovana kvadrokoptera+zavazi

Ac = [
0, 0, 0,                 0,                  0, 0,                  0,                  0, 1, 0, 0, 0, 0, 0, 0, 0;
0, 0, 0,                 0,                  0, 0,                  0,                  0, 0, 1, 0, 0, 0, 0, 0, 0;
0, 0, 0,                 0,                  0, 0,                  0,                  0, 0, 0, 1, 0, 0, 0, 0, 0;
0, 0, 0,                 0,                  0, 0,                  0,                  0, 0, 0, 0, 1, 0, 0, 0, 0;
0, 0, 0,                 0,                  0, 0,                  0,                  0, 0, 0, 0, 0, 1, 0, 0, 0;
0, 0, 0,                 0,                  0, 0,                  0,                  0, 0, 0, 0, 0, 0, 1, 0, 0;
0, 0, 0,                 0,                  0, 0,                  0,                  0, 0, 0, 0, 0, 0, 0, 1, 0;
0, 0, 0,                 0,                  0, 0,                  0,                  0, 0, 0, 0, 0, 0, 0, 0, 1;
0, 0, 0,                 0,      (g*(M + m))/M, 0,            (g*m)/M,                  0, 0, 0, 0, 0, 0, 0, 0, 0;
0, 0, 0,    -(g*(M + m))/M,                  0, 0,                  0,            (g*m)/M, 0, 0, 0, 0, 0, 0, 0, 0;
0, 0, 0,                 0,                  0, 0,                  0,                  0, 0, 0, 0, 0, 0, 0, 0, 0;
0, 0, 0,                 0,                  0, 0,                  0,                  0, 0, 0, 0, 0, 0, 0, 0, 0;
0, 0, 0,                 0,                  0, 0,                  0,                  0, 0, 0, 0, 0, 0, 0, 0, 0;
0, 0, 0,                 0,                  0, 0,                  0,                  0, 0, 0, 0, 0, 0, 0, 0, 0;
0, 0, 0,                 0, -(g*(M + m))/(M*d), 0, -(g*(M + m))/(M*d),                  0, 0, 0, 0, 0, 0, 0, 0, 0;
0, 0, 0, (g*(M + m))/(M*d),                  0, 0,                  0, -(g*(M + m))/(M*d), 0, 0, 0, 0, 0, 0, 0, 0];

== matlab function kopter_se_zavazim_state_feedback/Pozorovatel/Bc ==
  data: M parameter; Bc output; Ixx parameter; Iyy parameter; Izz parameter; m parameter
function Bc = fcn(M, Ixx, Iyy, Izz, m)
% Matice Ac linearizovana

Bc = [
        0,     0,     0,     0;
        0,     0,     0,     0;
        0,     0,     0,     0;
        0,     0,     0,     0;
        0,     0,     0,     0;
        0,     0,     0,     0;
        0,     0,     0,     0;
        0,     0,     0,     0;
        0,     0,     0,     0;
        0,     0,     0,     0;
1/(M + m),     0,     0,     0;
        0, 1/Ixx,     0,     0;
        0,     0, 1/Iyy,     0;
        0,     0,     0, 1/Izz;
        0,     0,     0,     0;
        0,     0,     0,     0];

== matlab function kopter_se_zavazim_state_feedback/u na (rad//s)^2 ==
  data: u input; wi output; b_moment parameter; k_thrust parameter; l parameter
function wi = fcn(u, b_moment, k_thrust, l)

T = u(1);
Tau_phi = u(2);
Tau_theta = u(3);
Tau_psi = u(4);

w1 = ( (Tau_phi*b_moment - Tau_theta*b_moment + l*T*b_moment + l*Tau_psi*k_thrust)/(4*l*b_moment*k_thrust));
w2 = ( (-Tau_theta*b_moment - Tau_phi*b_moment + l*T*b_moment - l*Tau_psi*k_thrust)/(4*l*b_moment*k_thrust));
w3 = ( (Tau_theta*b_moment - Tau_phi*b_moment + l*T*b_moment + l*Tau_psi*k_thrust)/(4*l*b_moment*k_thrust));
w4 = ( (Tau_phi*b_moment + Tau_theta*b_moment + l*T*b_moment - l*Tau_psi*k_thrust)/(4*l*b_moment*k_thrust));

wi = [w1;w2;w3;w4];
